simulink model "lab3_p1"  (R2020a)
settings: Solver=VariableStepAuto  StartTime=0.0  StopTime=stop_time  RelTol=1e-3
InitFcn:
  | % Read in the audio file
  | [input_wav_signal, Fs_in] = audioread('acoustic.wav');
  | % Fs_in = 11025, we need to convert this to Fs = 48k
  | 
  | % Convert the Sampling rate to 48 kHz
  | signal = resample(input_wav_signal, 48000, 11025);
  | Fs = 48000; % This is our desired sample rate that we converted to
  | Ts = 1/Fs; % The associated sample period
  | 
  | % Put signal inot a timeseries format
  | timevals = [0:length(signal)-1]*Ts;
  | input_signal = timeseries(signal,timevals);
  | 
  | % Set the simulation stop time
  | stop_time = length(signal)*Ts;
  | 
  | % Fixed-point precision we want the signal to be converted to
  | W_bits = 32;
  | F_bits = 28;
StopFcn:
  | y_out = output_signal.Data(:);
  | plot(y_out)
  | soundsc(y_out,Fs)
settings Model: Creator=Owner  LastModifiedBy=Owner
settings DataIOCC: ReturnWorkspaceOutputs=off

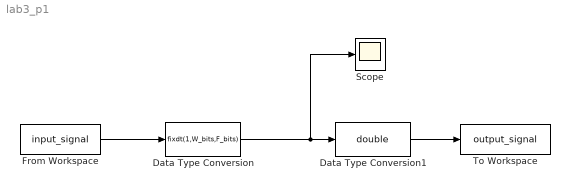
== system lab3_p1 ==
  Data Type Conversion : DataTypeConversion  OutDataTypeStr=fixdt(1,W_bits,F_bits)
  Data Type Conversion1 : DataTypeConversion  OutDataTypeStr=double
  From Workspace : FromWorkspace  VariableName=input_signal  SampleTime=Ts
  Scope : Scope
  To Workspace : ToWorkspace  VariableName=output_signal  SaveFormat=Timeseries  SampleTime=-1
  wires:
  From Workspace/1 -> Data Type Conversion/1
  Data Type Conversion/1 -> Scope/1, Data Type Conversion1/1
  Data Type Conversion1/1 -> To Workspace/1
